simulink model "SDRIP"  (R2022a)
settings: Solver=FixedStepDiscrete  StartTime=0.0  StopTime=simTime  RelTol=1e-3
values from neighbouring files (symbols this model uses):
  configuration = fi(1,0,2,0)    [main_testSDRIP.m]
  input = waveformTest    [main_testSDRIP.m]
  Nrepeat = 4    [main_testSDRIP.m]
  sequenceLength = numel(sequenceXcorr)    [main_testSDRIP.m]
  timerPC = 80    [main_testSDRIP.m]
  timerRX = 10    [main_testSDRIP.m]
  timerTX = 20    [main_testSDRIP.m]
libraries: dspsrcs4 x3, hdlsllib x1
settings Model: DataTypeOverride=Off  Creator=ASAHIN  LastModifiedBy=alpha
settings SolverCC: AlgebraicLoopSolver=TrustRegion
settings OptimizationCC: BlockReduction=off  ConditionallyExecuteInputs=off  DefaultParameterBehavior=Inlined  InheritOutputTypeSmallerThanSingle=on
settings DebuggingCC: AlgebraicLoopMsg=error  SingleTaskRateTransMsg=error  UnconnectedInputMsg=warning  UnconnectedOutputMsg=warning  UnconnectedLineMsg=warning  SFMachineParentedDataDiag=warning
settings HardwareCC: ProdBitPerPointer=32  ProdBitPerSizeT=32  ProdBitPerPtrDiffT=32  ProdLargestAtomicFloat=None  ProdIntDivRoundTo=Undefined  ProdEndianess=Unspecified  ProdWordSize=32  ProdHWDeviceType=ASIC/FPGA->ASIC/FPGA  TargetBitPerPointer=64  TargetBitPerSizeT=64  TargetBitPerPtrDiffT=64  TargetLongLongMode=on  TargetIntDivRoundTo=Zero  TargetEndianess=LittleEndian  TargetWordSize=64  TargetHWDeviceType=Custom Processor->MATLAB Host Computer  ProdEqTarget=off
settings RTWCC: DLArmComputeVersion=19.05

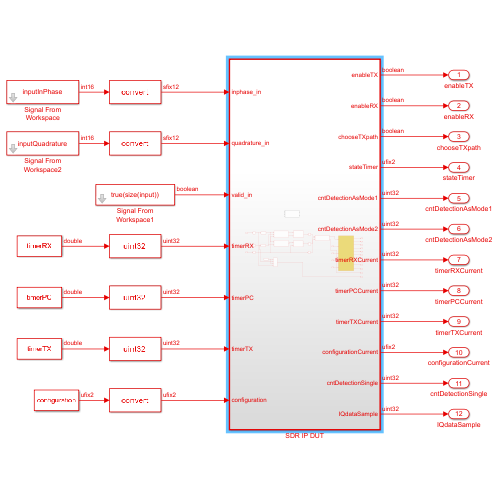
[thumbnail: Simulink's stored preview of the top-level diagram]
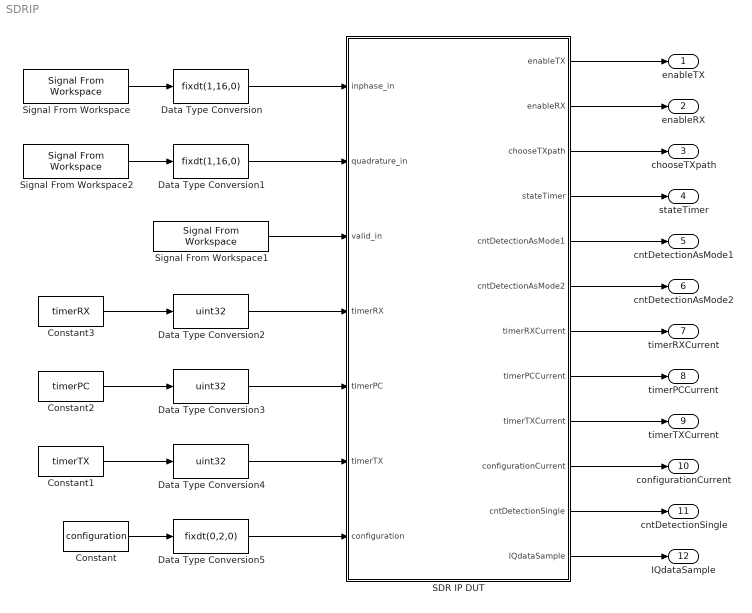
== system SDRIP ==
  Constant : Constant  Value=configuration  SampleTime=-1
  Constant1 : Constant  Value=timerTX  SampleTime=-1
  Constant2 : Constant  Value=timerPC  SampleTime=-1
  Constant3 : Constant  Value=timerRX  SampleTime=-1
  Data Type Conversion : DataTypeConversion  OutDataTypeStr=fixdt(1,16,0)  SaturateOnIntegerOverflow=off  RndMeth=Floor
  Data Type Conversion1 : DataTypeConversion  OutDataTypeStr=fixdt(1,16,0)  SaturateOnIntegerOverflow=off  RndMeth=Floor
  Data Type Conversion2 : DataTypeConversion  OutDataTypeStr=uint32  SaturateOnIntegerOverflow=off  RndMeth=Floor
  Data Type Conversion3 : DataTypeConversion  OutDataTypeStr=uint32  SaturateOnIntegerOverflow=off  RndMeth=Floor
  Data Type Conversion4 : DataTypeConversion  OutDataTypeStr=uint32  SaturateOnIntegerOverflow=off  RndMeth=Floor
  Data Type Conversion5 : DataTypeConversion  OutDataTypeStr=fixdt(0,2,0)  SaturateOnIntegerOverflow=off  RndMeth=Floor
  SDR IP DUT : Subsystem  TreatAsAtomicUnit=on
  Signal From Workspace : dspsrcs4/Signal From Workspace  X=inputInPhase  Ts=1  nsamps=1  OutputAfterFinalValue=Setting to zero  ignoreOrWarnInputAndFrameLengths=off  OutputFrames=off
  Signal From Workspace1 : dspsrcs4/Signal From Workspace  X=true(size(input))  Ts=1  nsamps=1  OutputAfterFinalValue=Setting to zero  ignoreOrWarnInputAndFrameLengths=off  OutputFrames=off
  Signal From Workspace2 : dspsrcs4/Signal From Workspace  X=inputQuadrature  Ts=1  nsamps=1  OutputAfterFinalValue=Setting to zero  ignoreOrWarnInputAndFrameLengths=off  OutputFrames=off
  enableTX : Outport
  enableRX : Outport  Port=2
  chooseTXpath : Outport  Port=3
  stateTimer : Outport  Port=4
  cntDetectionAsMode1 : Outport  Port=5
  cntDetectionAsMode2 : Outport  Port=6
  timerRXCurrent : Outport  Port=7
  timerPCCurrent : Outport  Port=8
  timerTXCurrent : Outport  Port=9
  configurationCurrent : Outport  Port=10
  cntDetectionSingle : Outport  Port=11
  IQdataSample : Outport  Port=12
  wires:
  SDR IP DUT/1(enableTX) -> enableTX/1
  SDR IP DUT/2(enableRX) -> enableRX/1
  Signal From Workspace2/1 -> Data Type Conversion1/1
  Signal From Workspace/1 -> Data Type Conversion/1
  Signal From Workspace1/1 -> SDR IP DUT/3(valid_in)
  Constant1/1 -> Data Type Conversion4/1
  Constant/1 -> Data Type Conversion5/1
  Data Type Conversion5/1 -> SDR IP DUT/7(configuration)
  Data Type Conversion1/1 -> SDR IP DUT/2(quadrature_in)
  Data Type Conversion/1 -> SDR IP DUT/1(inphase_in)
  Constant2/1 -> Data Type Conversion3/1
  Data Type Conversion3/1 -> SDR IP DUT/5(timerPC)
  SDR IP DUT/3(chooseTXpath) -> chooseTXpath/1
  Data Type Conversion4/1 -> SDR IP DUT/6(timerTX)
  Data Type Conversion2/1 -> SDR IP DUT/4(timerRX)
  Constant3/1 -> Data Type Conversion2/1
  SDR IP DUT/4(stateTimer) -> stateTimer/1
  SDR IP DUT/9(timerTXCurrent) -> timerTXCurrent/1
  SDR IP DUT/8(timerPCCurrent) -> timerPCCurrent/1
  SDR IP DUT/6(cntDetectionAsMode2) -> cntDetectionAsMode2/1
  SDR IP DUT/10(configurationCurrent) -> configurationCurrent/1
  SDR IP DUT/5(cntDetectionAsMode1) -> cntDetectionAsMode1/1
  SDR IP DUT/11(cntDetectionSingle) -> cntDetectionSingle/1
  SDR IP DUT/12(IQdataSample) -> IQdataSample/1
  SDR IP DUT/7(timerRXCurrent) -> timerRXCurrent/1

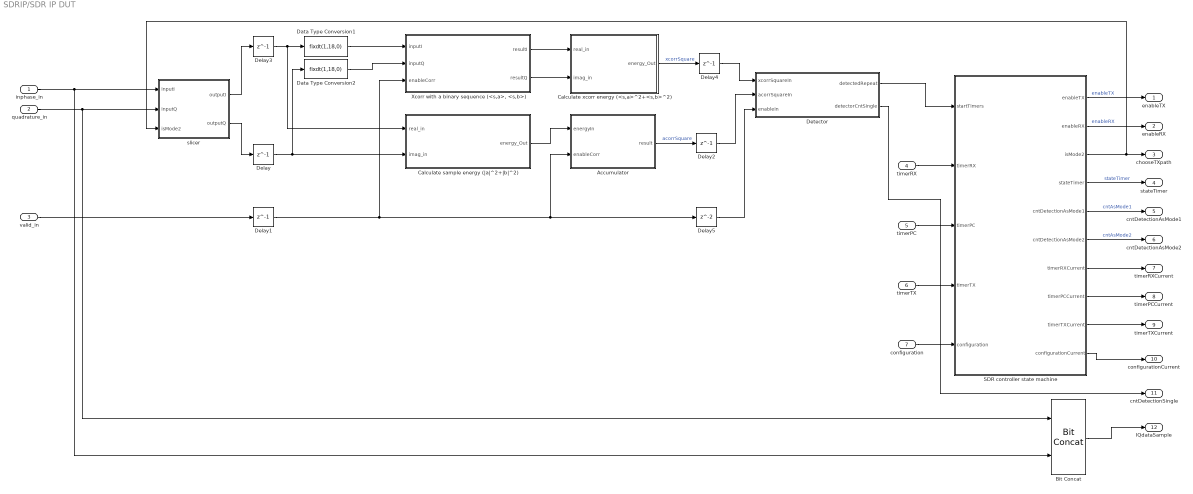
== system SDRIP/SDR IP DUT ==
  inphase_in : Inport
  quadrature_in : Inport  Port=2
  valid_in : Inport  Port=3
  timerRX : Inport  Port=4
  timerPC : Inport  Port=5
  timerTX : Inport  Port=6
  configuration : Inport  Port=7
  Accumulator : MATLAB Function  TreatAsAtomicUnit=on
  Bit Concat : hdlsllib/Logic and Bit Operations/Bit Concat  numInputs=2
  Calculate sample energy (|a|^2+|b|^2) : Subsystem
  Calculate xcorr energy (<s,a>^2+<s,b>^2) : Subsystem
  Data Type Conversion1 : DataTypeConversion  OutDataTypeStr=fixdt(1,18,0)  SaturateOnIntegerOverflow=off  RndMeth=Floor
  Data Type Conversion2 : DataTypeConversion  OutDataTypeStr=fixdt(1,18,0)  SaturateOnIntegerOverflow=off  RndMeth=Floor
  Delay{,1..4} (5 alike) : Delay  DelayLength=1  InitialCondition=0
  Delay5 : Delay  InitialCondition=0
  Detector : MATLAB Function  TreatAsAtomicUnit=on
  SDR controller state machine : MATLAB Function  TreatAsAtomicUnit=on
  "Xcorr with a binary sequence (<s,a>, <s,b>)" : MATLAB Function  TreatAsAtomicUnit=on
  slicer : MATLAB Function  TreatAsAtomicUnit=on
  enableTX : Outport
  enableRX : Outport  Port=2
  chooseTXpath : Outport  Port=3
  stateTimer : Outport  Port=4
  cntDetectionAsMode1 : Outport  Port=5
  cntDetectionAsMode2 : Outport  Port=6
  timerRXCurrent : Outport  Port=7
  timerPCCurrent : Outport  Port=8
  timerTXCurrent : Outport  Port=9
  configurationCurrent : Outport  Port=10
  cntDetectionSingle : Outport  Port=11
  IQdataSample : Outport  Port=12
  wires:
  "Xcorr with a binary sequence (<s,a>, <s,b>)"/1(resultI) -> Calculate xcorr energy (<s,a>^2+<s,b>^2)/1(real_in)
  Calculate xcorr energy (<s,a>^2+<s,b>^2)/1(energy_Out) -> Delay4/1  "xcorrSquare"
  Detector/1(detectedRepeat) -> SDR controller state machine/1(startTimers)
  timerRX/1 -> SDR controller state machine/2(timerRX)
  timerPC/1 -> SDR controller state machine/3(timerPC)
  timerTX/1 -> SDR controller state machine/4(timerTX)
  configuration/1 -> SDR controller state machine/5(configuration)
  SDR controller state machine/1(enableTX) -> enableTX/1  "enableTX"
  SDR controller state machine/2(enableRX) -> enableRX/1  "enableRX"
  SDR controller state machine/3(isMode2) -> slicer/3(isMode2), chooseTXpath/1
  SDR controller state machine/4(stateTimer) -> stateTimer/1  "stateTimer"
  SDR controller state machine/5(cntDetectionAsMode1) -> cntDetectionAsMode1/1  "cntAsMode1"
  SDR controller state machine/6(cntDetectionAsMode2) -> cntDetectionAsMode2/1  "cntAsMode2"
  SDR controller state machine/7(timerRXCurrent) -> timerRXCurrent/1
  SDR controller state machine/8(timerPCCurrent) -> timerPCCurrent/1
  SDR controller state machine/9(timerTXCurrent) -> timerTXCurrent/1
  SDR controller state machine/10(configurationCurrent) -> configurationCurrent/1
  Data Type Conversion1/1 -> "Xcorr with a binary sequence (<s,a>, <s,b>)"/1(inputI)
  Delay1/1 -> "Xcorr with a binary sequence (<s,a>, <s,b>)"/3(enableCorr), Delay5/1, Accumulator/2(enableCorr)
  quadrature_in/1 -> Bit Concat/1, slicer/2(inputQ)
  Data Type Conversion2/1 -> "Xcorr with a binary sequence (<s,a>, <s,b>)"/2(inputQ)
  "Xcorr with a binary sequence (<s,a>, <s,b>)"/2(resultQ) -> Calculate xcorr energy (<s,a>^2+<s,b>^2)/2(imag_in)
  inphase_in/1 -> Bit Concat/2, slicer/1(inputI)
  Calculate sample energy (|a|^2+|b|^2)/1(energy_Out) -> Accumulator/1(energyIn)
  Accumulator/1(result) -> Delay2/1  "acorrSquare"
  valid_in/1 -> Delay1/1
  Delay4/1 -> Detector/1(xcorrSquareIn)
  Delay/1 -> Calculate sample energy (|a|^2+|b|^2)/2(imag_in), Data Type Conversion2/1
  Delay3/1 -> Calculate sample energy (|a|^2+|b|^2)/1(real_in), Data Type Conversion1/1
  Detector/2(detectorCntSingle) -> cntDetectionSingle/1
  Delay5/1 -> Detector/3(enableIn)
  Bit Concat/1 -> IQdataSample/1
  slicer/1(outputI) -> Delay3/1
  slicer/2(outputQ) -> Delay/1
  Delay2/1 -> Detector/2(acorrSquareIn)

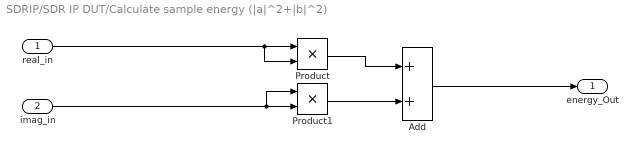
== system SDRIP/SDR IP DUT/Calculate sample energy (|a|^2+|b|^2) ==
  real_in : Inport
  imag_in : Inport  Port=2
  Add : Sum  AccumDataTypeStr=fixdt(0,25,0)
  Product : Product  OutDataTypeStr=fixdt(0,24,0)
  Product1 : Product  OutDataTypeStr=fixdt(0,24,0)
  energy_Out : Outport
  wires:
  imag_in/1 -> Product1/1, Product1/2
  Product1/1 -> Add/2
  real_in/1 -> Product/2, Product/1
  Add/1 -> energy_Out/1
  Product/1 -> Add/1

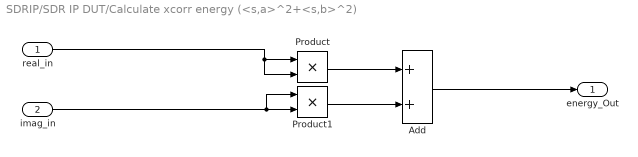
== system SDRIP/SDR IP DUT/Calculate xcorr energy (<s,a>^2+<s,b>^2) ==
  real_in : Inport
  imag_in : Inport  Port=2
  Add : Sum
  Product : Product  OutDataTypeStr=fixdt(0,36,0)
  Product1 : Product  OutDataTypeStr=fixdt(0,36,0)
  energy_Out : Outport
  wires:
  imag_in/1 -> Product1/1, Product1/2
  Product1/1 -> Add/2
  real_in/1 -> Product/2, Product/1
  Add/1 -> energy_Out/1
  Product/1 -> Add/1

== matlab function SDRIP/SDR IP DUT/SDR controller state machine ==
  settings: updateMethod=DISCRETE  fimath=fimath('RoundingMethod', 'Floor','OverflowAction', 'Wrap','ProductMode', 'FullPrecision', 'SumMode', 'FullPrecision')
  data: startTimers input; timerRX input; timerPC input; timerTX input; configuration input; enableTX output; enableRX output; isMode2 output; stateTimer output; cntDetectionAsMode1 output; cntDetectionAsMode2 output; timerRXCurrent output; timerPCCurrent output; timerTXCurrent output; configurationCurrent output
function [enableTX, enableRX, isMode2, stateTimer, cntDetectionAsMode1, cntDetectionAsMode2,  timerRXCurrent, timerPCCurrent, timerTXCurrent, configurationCurrent] = fcn_SDRController(startTimers, timerRX, timerPC, timerTX, configuration)
    %% Initialize Registers
    persistent cntMode1_reg;
    if isempty(cntMode1_reg)
        cntMode1_reg = uint32(0);
    end
    persistent cntMode2_reg;
    if isempty(cntMode2_reg)
        cntMode2_reg = uint32(0);
    end    
    persistent TimerState_reg;
    if isempty(TimerState_reg)
        TimerState_reg = fi(0,0,2,0);
    end    
    persistent timerRX_reg;
    if isempty(timerRX_reg)
        timerRX_reg = uint32(512);
    end
    persistent timerPC_reg;
    if isempty(timerPC_reg)
        timerPC_reg = uint32(512);
    end    
    persistent timerTX_reg;
    if isempty(timerTX_reg)
        timerTX_reg = uint32(512);
    end     
    persistent configuration_reg;
    if isempty(configuration_reg)
        configuration_reg = fi(0,0,2,0) ;
    end  

    persistent startTimers_reg;
    if isempty(startTimers_reg)
        startTimers_reg = false;
    end  

    %% Set outputs
    isMode2 = configuration_reg == fi(2,0,2,0);
    cntDetectionAsMode1 = cntMode1_reg;
    cntDetectionAsMode2 = cntMode2_reg;
    timerRXCurrent = timerRX_reg;
    timerTXCurrent = timerTX_reg;
    timerPCCurrent = timerPC_reg;
    configurationCurrent = configuration_reg;
    stateTimer = TimerState_reg;

    if configuration_reg==fi(1,0,2,0)
        enableRX = TimerState_reg==fi(1,0,2,0); 
        enableTX = TimerState_reg==fi(3,0,2,0);
    elseif configuration_reg==fi(2,0,2,0)
        enableRX = TimerState_reg~=fi(2,0,2,0);
        enableTX = true;
    else
        enableRX = true;
        enableTX = true;
    end

    
    %% Update Registers
    switch TimerState_reg
        case 0
            timerRX_reg = timerRX;
            timerPC_reg = timerPC;
            timerTX_reg = timerTX;
            if configuration_reg == fi(1,0,2,0) && startTimers_reg == true
                TimerState_reg = fi(1,0,2,0) ;
                cntMode1_reg = cntMode1_reg + 1;
            elseif configuration_reg == fi(2,0,2,0)  && startTimers_reg == true
                TimerState_reg = fi(2,0,2,0) ;
                cntMode2_reg = cntMode2_reg + 1;
            end
        case 1
            if timerRX_reg == fi(0,0,2,0) 
                TimerState_reg = fi(2,0,2,0) ;            
            else
                timerRX_reg = timerRX_reg - 1;
            end
        case 2
            if timerPC_reg == fi(0,0,2,0) 
                if configuration_reg==fi(1,0,2,0)
                    TimerState_reg = fi(3,0,2,0) ;
                elseif configuration_reg==fi(2,0,2,0)
                    TimerState_reg = fi(0,0,2,0) ;
                end   
            else
                timerPC_reg = timerPC_reg - 1;
            end
        case 3
            if timerTX_reg == fi(0,0,2,0) 
                TimerState_reg = fi(0,0,2,0) ;
            else
                timerTX_reg = timerTX_reg - 1;
            end
    end
    configuration_reg = configuration;
    startTimers_reg = startTimers;
end

== matlab function SDRIP/SDR IP DUT/Detector ==
  settings: fimath=fimath('RoundingMethod', 'Floor','OverflowAction', 'Wrap','ProductMode', 'FullPrecision', 'SumMode', 'FullPrecision')
  data: xcorrSquareIn input; detectedRepeat output; acorrSquareIn input; enableIn input; sequenceLength parameter; Nrepeat parameter; detectorCntSingle output
function [detectedRepeat,detectorCntSingle]  = fcn_comparator(xcorrSquareIn, acorrSquareIn, enableIn, sequenceLength, Nrepeat)
nbits = ceil(log2(sequenceLength));
indices = 2^nbits*[0:Nrepeat-1]+1;

persistent detectionHistory;
if isempty(detectionHistory)
    detectionHistory = fi(zeros((Nrepeat-1)*2^nbits+1,1),0,1,0);
end

persistent detectorCntSingle_reg;
if isempty(detectorCntSingle_reg)
    detectorCntSingle_reg = uint32(0);
end 


if  bitsra(xcorrSquareIn,nbits-2) >  acorrSquareIn 
    detected = true;
else
    detected = false;
end

detectedRepeat = all(detectionHistory(indices) == true);
detectorCntSingle = detectorCntSingle_reg;


if enableIn == true
    if detected == true
        detectorCntSingle_reg = detectorCntSingle_reg+1;
    end
    detectionHistory = [detected; detectionHistory(1:end-1)];
end

== matlab function SDRIP/SDR IP DUT/Xcorr with a binary sequence (<s,a>, <s,b>) ==
  settings: fimath=fimath('RoundingMethod', 'Floor','OverflowAction', 'Wrap','ProductMode', 'FullPrecision', 'SumMode', 'FullPrecision')
  data: inputI input; inputQ input; resultI output; sequenceXcorr parameter; enableCorr input; resultQ output
function [resultI, resultQ]= fcn_xcorr(inputI, inputQ, sequenceXcorr, enableCorr)
    numberOfBitsXcorrResult = 18;
    sequenceLength = numel(sequenceXcorr);

    %% Registers
    persistent delayOutputsI;
    if isempty(delayOutputsI)
        delayOutputsI = fi(zeros(sequenceLength,1),1,numberOfBitsXcorrResult,0);
    end

    persistent delayOutputsQ;
    if isempty(delayOutputsQ)
        delayOutputsQ = fi(zeros(sequenceLength,1),1,numberOfBitsXcorrResult,0);
    end    

    %% Set outputs
    resultI = delayOutputsI(end); 
    resultQ = delayOutputsQ(end); 
    
    %% Update registers
    sumsResultsI = fi(zeros(sequenceLength-1,1),1,numberOfBitsXcorrResult,0);
    inputINegated = -inputI;
    if sequenceXcorr(1) == true
        inputIP = inputI;
    else
        inputIP = inputINegated;
    end
    for indSumResult = 1:sequenceLength-1
        if sequenceXcorr(indSumResult+1) == true
            sumsResultsI(indSumResult) = delayOutputsI(indSumResult)+inputI;
        else
            sumsResultsI(indSumResult) = delayOutputsI(indSumResult)+inputINegated;
        end
    end

    sumsResultsQ = fi(zeros(sequenceLength-1,1),1,numberOfBitsXcorrResult,0);
    inputQNegated = -inputQ;
    if sequenceXcorr(1) == true
        inputQP = inputQ;
    else
        inputQP = inputQNegated;
    end
    for indSumResult = 1:sequenceLength-1
        if sequenceXcorr(indSumResult+1) == true
            sumsResultsQ(indSumResult) = delayOutputsQ(indSumResult)+inputQ;
        else
            sumsResultsQ(indSumResult) = delayOutputsQ(indSumResult)+inputQNegated;
        end
    end    

    if enableCorr == 1
        delayOutputsI = [inputIP; sumsResultsI];
        delayOutputsQ = [inputQP; sumsResultsQ];
    end
end

== matlab function SDRIP/SDR IP DUT/Accumulator ==
  settings: fimath=fimath('RoundingMethod', 'Floor','OverflowAction', 'Wrap','ProductMode', 'FullPrecision', 'SumMode', 'FullPrecision')
  data: energyIn input; result output; enableCorr input; sequenceLength parameter
function result = fcn_accumulator(energyIn, enableCorr, sequenceLength)
    numberOfBitsEnergy = 31;
    numberOfBitsDelay = 25;

    %% Registers
    persistent delayOutputs;
    if isempty(delayOutputs)
        delayOutputs = fi(zeros(sequenceLength,1),0,numberOfBitsDelay,0);
    end
    persistent energy;
    if isempty(energy)
        energy = fi(0,0,numberOfBitsEnergy,0);
    end

    %energyIn = fi(energyIn,0,numberOfBitsDelay,0,'RoundingMethod','floor', 'SumMode','FullPrecision','ProductMode','FullPrecision'); 

    %% Set outputs
    result = energy; 
    
    %% Update registers
    energyOut = delayOutputs(end);
    if enableCorr == 1
        delayOutputs(2:end) = delayOutputs(1:end-1);
        delayOutputs(1) = energyIn;
        aa = fi(energy,0,numberOfBitsEnergy-2,0) + energyIn - energyOut; % Full implementation
        energy = aa;
    end
end

== matlab function SDRIP/SDR IP DUT/slicer ==
  settings: fimath=fimath('RoundingMethod', 'Floor','OverflowAction', 'Wrap','ProductMode', 'FullPrecision', 'SumMode', 'FullPrecision')
  data: inputI input; inputQ input; outputI output; outputQ output; isMode2 input
function [outputI, outputQ]= fcn_slicer(inputI, inputQ, isMode2)
    inputIc = fi(inputI,1,16,0);
    inputQc = fi(inputQ,1,16,0);
    if isMode2 == false
        outputIc = bitsliceget(inputIc,12,1);
        outputQc = bitsliceget(inputQc,12,1);
    else
        outputIc = bitsliceget(inputIc,16,5);
        outputQc = bitsliceget(inputQc,16,5);
    end
    outputI = fi(outputIc,1,12,0);
    outputQ = fi(outputQc,1,12,0);    
end
